simulink model "MRAC"  (R2018b)
settings: Solver=VariableStepAuto  StartTime=0.0  StopTime=30  RelTol=1e-3
settings Model: Creator=Aslesh  LastModifiedBy=Aslesh

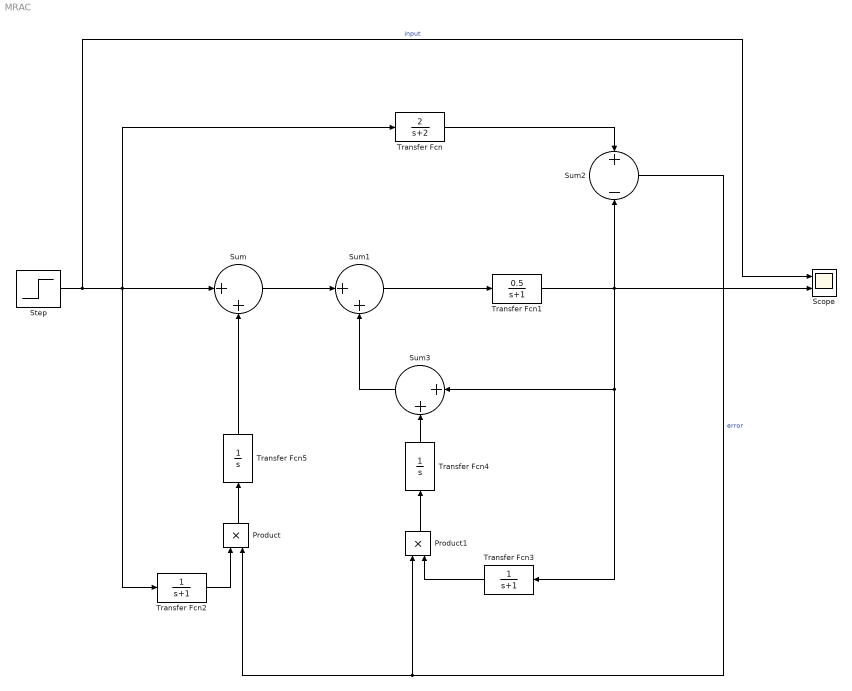
== system MRAC ==
  Product : Product
  Product1 : Product
  Scope : Scope  NumInputPorts=2
  Step : Step  SampleTime=0
  Sum : Sum  Inputs=|++
  Sum1 : Sum  Inputs=|++
  Sum2 : Sum  Inputs=+|-
  Sum3 : Sum  Inputs=|++
  Transfer Fcn : TransferFcn  Numerator=[2]  Denominator=[1 2]
  Transfer Fcn1 : TransferFcn  Numerator=[0.5]  Denominator=[1 1]
  Transfer Fcn2 : TransferFcn  Denominator=[1 1]
  Transfer Fcn3 : TransferFcn  Denominator=[1 1]
  Transfer Fcn4 : TransferFcn  Denominator=[1 0]
  Transfer Fcn5 : TransferFcn  Denominator=[1 0]
  wires:
  Sum/1 -> Sum1/1
  Sum1/1 -> Transfer Fcn1/1
  Transfer Fcn1/1 -> Transfer Fcn3/1, Sum3/1, Sum2/2, Scope/2
  Transfer Fcn/1 -> Sum2/1
  Step/1 -> Transfer Fcn2/1, Transfer Fcn/1, Sum/1, Scope/1  "input"
  Transfer Fcn5/1 -> Sum/2
  Product/1 -> Transfer Fcn5/1
  Sum2/1 -> Product1/1, Product/2  "error"
  Transfer Fcn2/1 -> Product/1
  Sum3/1 -> Sum1/2
  Transfer Fcn4/1 -> Sum3/2
  Product1/1 -> Transfer Fcn4/1
  Transfer Fcn3/1 -> Product1/2
